simulink model "obserwator_regulator_odstanu_niemierzone"  (R2023a)
settings: Solver=VariableStepAuto  StartTime=0.0  StopTime=10  RelTol=1e-3
values from neighbouring files (symbols this model uses):
  K = acker(A, B, [sb, sb, sb])    [do_workspace.m]    (also in zadania_1_5.m)
  L = acker(A', C', [s0, s0, s0])    [do_workspace.m]    (also in zadania_1_5.m)
settings Model: Creator=adams  LastModifiedBy=adams

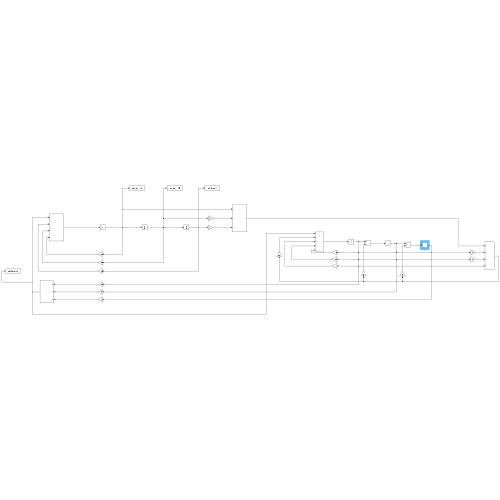
[thumbnail: Simulink's stored preview of the top-level diagram]
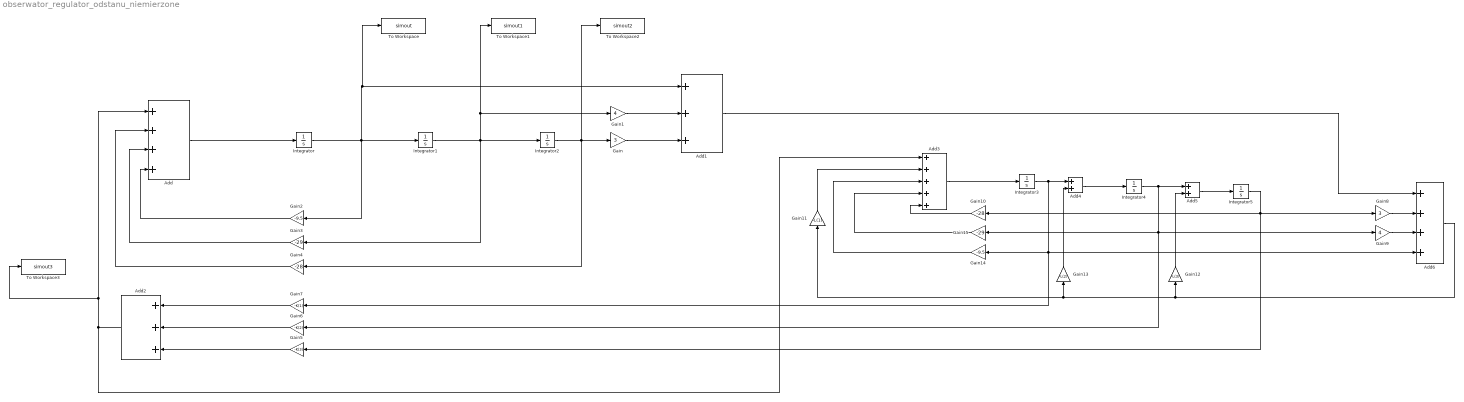
== system obserwator_regulator_odstanu_niemierzone ==
  Add : Sum  Inputs=++++
  Add1 : Sum  Inputs=+++
  Add2 : Sum  Inputs=+++
  Add3 : Sum  Inputs=+++++
  Add4 : Sum
  Add5 : Sum
  Add6 : Sum  Inputs=++++
  Gain : Gain  Gain=3
  Gain1 : Gain  Gain=4
  Gain10 : Gain  Gain=-28
  Gain11 : Gain  Gain=-L(1)
  Gain12 : Gain  Gain=-L(3)
  Gain13 : Gain  Gain=-L(2)
  Gain14 : Gain  Gain=-9.5
  Gain15 : Gain  Gain=-29
  Gain2 : Gain  Gain=-9.5
  Gain3 : Gain  Gain=-29
  Gain4 : Gain  Gain=-28
  Gain5 : Gain  Gain=-K(3)
  Gain6 : Gain  Gain=-K(2)
  Gain7 : Gain  Gain=-K(1)
  Gain8 : Gain  Gain=3
  Gain9 : Gain  Gain=4
  Integrator : Integrator  InitialCondition=-1
  Integrator1 : Integrator  InitialCondition=-1
  Integrator2 : Integrator  InitialCondition=2
  Integrator3 : Integrator  InitialCondition=10
  Integrator4 : Integrator  InitialCondition=20
  Integrator5 : Integrator  InitialCondition=30
  To Workspace : ToWorkspace  VariableName=simout  SaveFormat=Structure With Time  SampleTime=-1
  To Workspace1 : ToWorkspace  VariableName=simout1  SaveFormat=Structure With Time  SampleTime=-1
  To Workspace2 : ToWorkspace  VariableName=simout2  SaveFormat=Structure With Time  SampleTime=-1
  To Workspace3 : ToWorkspace  VariableName=simout3  SaveFormat=Structure With Time  SampleTime=-1
  wires:
  Integrator5/1 -> Gain5/1, Gain8/1, Gain10/1
  Integrator2/1 -> To Workspace2/1, Gain4/1, Gain/1
  Gain10/1 -> Add3/5
  Add1/1 -> Add6/1
  Integrator1/1 -> To Workspace1/1, Gain1/1, Integrator2/1, Gain3/1
  Gain4/1 -> Add/2
  Gain1/1 -> Add1/2
  Gain13/1 -> Add4/2
  Add2/1 -> To Workspace3/1, Add/1, Add3/1
  Gain3/1 -> Add/3
  Gain6/1 -> Add2/2
  Gain11/1 -> Add3/2
  Add5/1 -> Integrator5/1
  Gain12/1 -> Add5/2
  Gain14/1 -> Add3/3
  Add4/1 -> Integrator4/1
  Gain5/1 -> Add2/3
  Integrator3/1 -> Gain7/1, Gain14/1, Add6/4, Add4/1
  Gain9/1 -> Add6/3
  Add/1 -> Integrator/1
  Gain15/1 -> Add3/4
  Gain2/1 -> Add/4
  Gain/1 -> Add1/3
  Gain7/1 -> Add2/1
  Integrator/1 -> Gain2/1, To Workspace/1, Add1/1, Integrator1/1
  Add6/1 -> Gain13/1, Gain11/1, Gain12/1
  Gain8/1 -> Add6/2
  Add3/1 -> Integrator3/1
  Integrator4/1 -> Gain6/1, Gain15/1, Gain9/1, Add5/1
